simulink model "PositionControl_trajectory_obs"  (R2019a)
settings: Solver=ode3  StartTime=0.0  StopTime=100.0  FixedStep=Ts  RelTol=1e-3
values from neighbouring files (symbols this model uses):
  error_margin = 0.05    [Control_borroso_obstaculo_reference.m]    (also in Control_borroso_obstaculo_trajectory.m = 0)
  obsx = 3    [Control_borroso_obstaculo_reference.m]    (also in Control_borroso_obstaculo_trajectory.m = 2)
  obsy = 3    [Control_borroso_obstaculo_reference.m]    (also in Control_borroso_obstaculo_trajectory.m = 1)
  th_0 = w0    (= 0)    [Control_borroso_obstaculo_trajectory.m]
  Ts = 100e-3    (= 0.1)    [Control_borroso_obstaculo_reference.m]    (also in Control_borroso_obstaculo_trajectory.m)
  w0 = pi/2    (= 1.57079632679)    [Control_borroso_obstaculo_reference.m]    (also in Control_borroso_obstaculo_trajectory.m = 0)
  x0 = 0    [Control_borroso_obstaculo_reference.m]    (also in Control_borroso_obstaculo_trajectory.m = -5)
  x_0 = 0    [Control_borroso_obstaculo_trajectory.m]
  y0 = 0    [Control_borroso_obstaculo_reference.m]    (also in Control_borroso_obstaculo_trajectory.m)
  y_0 = y0    (= 0)    [Control_borroso_obstaculo_trajectory.m]
undefined symbols (not defined in the file or in its folder): DiscIntNeverNeededParam, sigbuilder_block
libraries: fuzblock x1, simulink x1
settings Model: Creator=mrblissfulgrin  LastModifiedBy=juanjosecordoba
settings DataIOCC: ReturnWorkspaceOutputs=off

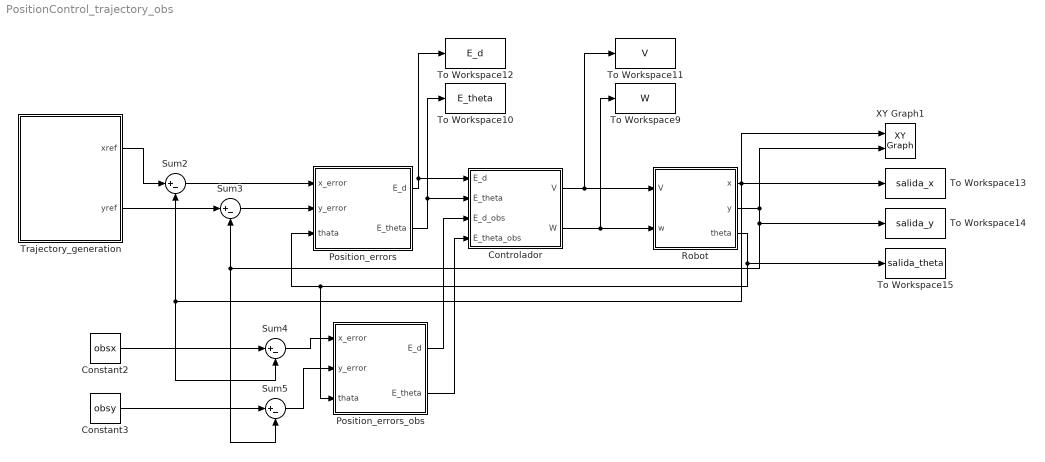
== system PositionControl_trajectory_obs ==
  Constant2 : Constant  Value=obsx  SampleTime=Ts
  Constant3 : Constant  Value=obsy  SampleTime=Ts
  Controlador : Subsystem
  Position_errors : Subsystem
  Position_errors_obs : Subsystem
  Robot : Subsystem
  Sum{2..5} (4 alike) : Sum  Inputs=|+-
  To Workspace10 : ToWorkspace  VariableName=E_theta  SaveFormat=Structure With Time  SampleTime=Ts
  To Workspace11 : ToWorkspace  VariableName=V  SaveFormat=Structure With Time  SampleTime=Ts
  To Workspace12 : ToWorkspace  VariableName=E_d  SaveFormat=Structure With Time  SampleTime=Ts
  To Workspace13 : ToWorkspace  VariableName=salida_x  SaveFormat=Structure With Time  SampleTime=Ts
  To Workspace14 : ToWorkspace  VariableName=salida_y  SaveFormat=Structure With Time  SampleTime=Ts
  To Workspace15 : ToWorkspace  VariableName=salida_theta  SaveFormat=Structure With Time  SampleTime=Ts
  To Workspace9 : ToWorkspace  VariableName=W  SaveFormat=Structure With Time  SampleTime=Ts
  Trajectory_generation : Subsystem
  XY Graph1 : simulink/Sinks/XY Graph  xmin=-10  xmax=10  ymin=-10  ymax=10  st=Ts
  wires:
  Constant3/1 -> Sum5/1
  Controlador/1("V ") -> Robot/1(V), To Workspace11/1
  Position_errors_obs/1(E_d) -> Controlador/3(E_d_obs)
  Position_errors/2(E_theta) -> To Workspace10/1, Controlador/2(E_theta)
  Trajectory_generation/2(yref) -> Sum3/1
  Constant2/1 -> Sum4/1
  Sum4/1 -> Position_errors_obs/1(x_error)
  Sum5/1 -> Position_errors_obs/2(y_error)
  Robot/3(theta) -> To Workspace15/1, Position_errors_obs/3(thata), Position_errors/3(thata)
  Controlador/2(W) -> To Workspace9/1, Robot/2(w)
  Robot/2(y) -> To Workspace14/1, Sum3/2, Sum5/2, XY Graph1/2
  Position_errors/1(E_d) -> Controlador/1("E_d "), To Workspace12/1
  Position_errors_obs/2(E_theta) -> Controlador/4(E_theta_obs)
  Robot/1(x) -> XY Graph1/1, To Workspace13/1, Sum4/2, Sum2/2
  Sum3/1 -> Position_errors/2(y_error)
  Trajectory_generation/1(xref) -> Sum2/1
  Sum2/1 -> Position_errors/1(x_error)

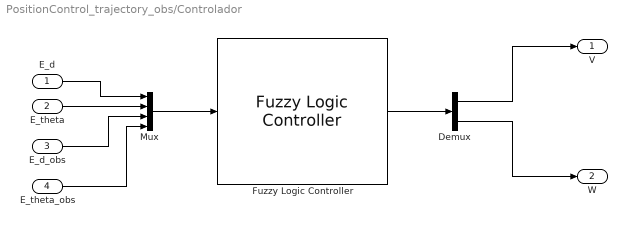
== system PositionControl_trajectory_obs/Controlador ==
  "E_d " : Inport  SampleTime=Ts
  E_theta : Inport  Port=2  SampleTime=Ts
  E_d_obs : Inport  Port=3  SampleTime=Ts
  E_theta_obs : Inport  Port=4  SampleTime=Ts
  Demux : Demux  Outputs=2
  Fuzzy Logic Controller : fuzblock/Fuzzy Logic  Controller  FIS=fis_name  OutputSampleNumber=101  DataType=double  FuzzifiedInputs=off  RuleFiringStrengths=off  RuleOutputs=off  AggregatedOutputs=off  SimulateUsing=Interpreted execution  OutOfRangeInputValueMessage=warning  NoRuleFiredMessage=warning  EmptyOutputFuzzySetMessage=warning
  Mux : Mux
  "V " : Outport  SampleTime=Ts
  W : Outport  Port=2  SampleTime=Ts
  wires:
  Demux/1 -> "V "/1
  Demux/2 -> W/1
  E_theta/1 -> Mux/2
  Mux/1 -> Fuzzy Logic Controller/1
  Fuzzy Logic Controller/1 -> Demux/1
  "E_d "/1 -> Mux/1
  E_d_obs/1 -> Mux/3
  E_theta_obs/1 -> Mux/4

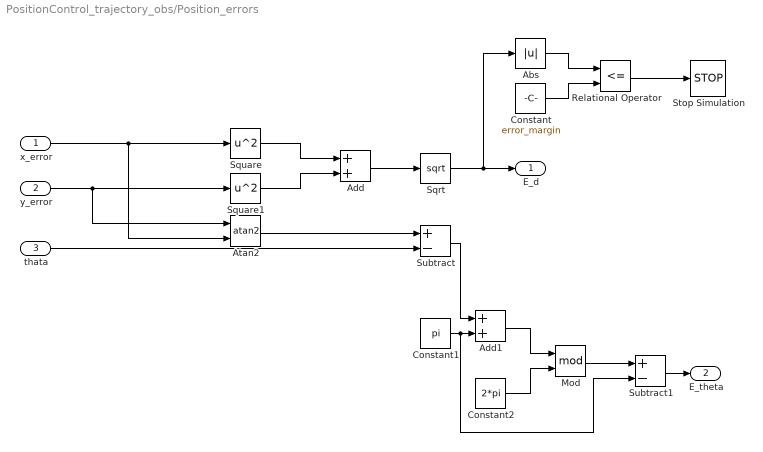
== system PositionControl_trajectory_obs/Position_errors ==
  x_error : Inport  SampleTime=Ts
  y_error : Inport  Port=2  SampleTime=Ts
  thata : Inport  Port=3  SampleTime=Ts
  Abs : Abs
  Add : Sum
  Add1 : Sum
  Atan2 : Trigonometry  Operator=atan2
  Constant : Constant  Value=error_margin  SampleTime=Ts
  Constant1 : Constant  Value=pi  SampleTime=Ts
  Constant2 : Constant  Value=2*pi
  Mod : Math  Operator=mod  SaturateOnIntegerOverflow=on
  Relational Operator : RelationalOperator  Operator=<=  OutDataTypeStr=boolean  RndMeth=Simplest
  Sqrt : Sqrt  SaturateOnIntegerOverflow=on
  Square : Math  Operator=square  SaturateOnIntegerOverflow=on
  Square1 : Math  Operator=square  SaturateOnIntegerOverflow=on
  Stop Simulation : Stop
  Subtract : Sum  Inputs=+-
  Subtract1 : Sum  Inputs=+-
  E_d : Outport  SampleTime=Ts
  E_theta : Outport  Port=2  SampleTime=Ts
  wires:
  Square/1 -> Add/1
  y_error/1 -> Square1/1, Atan2/1
  Add/1 -> Sqrt/1
  Square1/1 -> Add/2
  thata/1 -> Subtract/2
  x_error/1 -> Square/1, Atan2/2
  Subtract/1 -> Add1/1
  Atan2/1 -> Subtract/1
  Constant1/1 -> Subtract1/2, Add1/2
  Add1/1 -> Mod/1
  Constant2/1 -> Mod/2
  Mod/1 -> Subtract1/1
  Subtract1/1 -> E_theta/1
  Constant/1 -> Relational Operator/2
  Abs/1 -> Relational Operator/1
  Sqrt/1 -> Abs/1, E_d/1
  Relational Operator/1 -> Stop Simulation/1

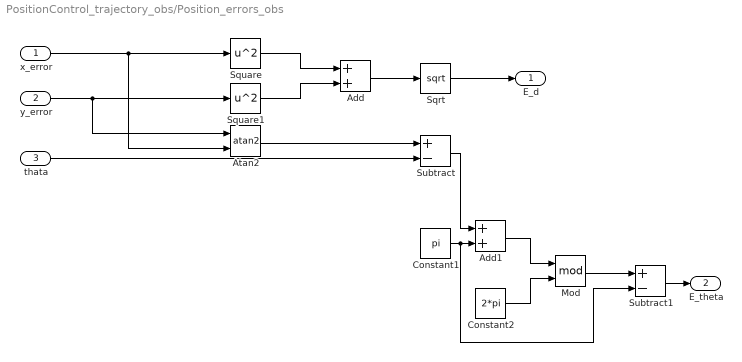
== system PositionControl_trajectory_obs/Position_errors_obs ==
  x_error : Inport  SampleTime=Ts
  y_error : Inport  Port=2  SampleTime=Ts
  thata : Inport  Port=3  SampleTime=Ts
  Add : Sum
  Add1 : Sum
  Atan2 : Trigonometry  Operator=atan2
  Constant1 : Constant  Value=pi  SampleTime=Ts
  Constant2 : Constant  Value=2*pi
  Mod : Math  Operator=mod  SaturateOnIntegerOverflow=on
  Sqrt : Sqrt  SaturateOnIntegerOverflow=on
  Square : Math  Operator=square  SaturateOnIntegerOverflow=on
  Square1 : Math  Operator=square  SaturateOnIntegerOverflow=on
  Subtract : Sum  Inputs=+-
  Subtract1 : Sum  Inputs=+-
  E_d : Outport  SampleTime=Ts
  E_theta : Outport  Port=2  SampleTime=Ts
  wires:
  Square/1 -> Add/1
  Sqrt/1 -> E_d/1
  y_error/1 -> Square1/1, Atan2/1
  Add/1 -> Sqrt/1
  Square1/1 -> Add/2
  thata/1 -> Subtract/2
  x_error/1 -> Square/1, Atan2/2
  Subtract/1 -> Add1/1
  Atan2/1 -> Subtract/1
  Constant1/1 -> Subtract1/2, Add1/2
  Add1/1 -> Mod/1
  Constant2/1 -> Mod/2
  Mod/1 -> Subtract1/1
  Subtract1/1 -> E_theta/1

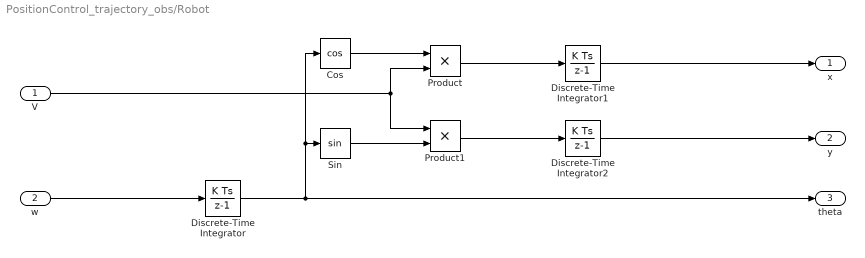
== system PositionControl_trajectory_obs/Robot ==
  V : Inport  SampleTime=Ts
  w : Inport  Port=2  SampleTime=Ts
  Cos : Trigonometry  Operator=cos
  Discrete-Time Integrator : DiscreteIntegrator  InitialCondition=w0  SampleTime=Ts  ICPrevOutput=DiscIntNeverNeededParam  ICPrevScaledInput=DiscIntNeverNeededParam
  Discrete-Time Integrator1 : DiscreteIntegrator  InitialCondition=x0  SampleTime=Ts  ICPrevOutput=DiscIntNeverNeededParam  ICPrevScaledInput=DiscIntNeverNeededParam
  Discrete-Time Integrator2 : DiscreteIntegrator  InitialCondition=y0  SampleTime=Ts  ICPrevOutput=DiscIntNeverNeededParam  ICPrevScaledInput=DiscIntNeverNeededParam
  Product : Product
  Product1 : Product
  Sin : Trigonometry
  x : Outport  SampleTime=Ts
  y : Outport  Port=2  SampleTime=Ts
  theta : Outport  Port=3  SampleTime=Ts
  wires:
  Discrete-Time Integrator2/1 -> y/1
  Product1/1 -> Discrete-Time Integrator2/1
  Cos/1 -> Product/1
  Sin/1 -> Product1/2
  w/1 -> Discrete-Time Integrator/1
  Discrete-Time Integrator1/1 -> x/1
  Product/1 -> Discrete-Time Integrator1/1
  V/1 -> Product/2, Product1/1
  Discrete-Time Integrator/1 -> theta/1, Sin/1, Cos/1

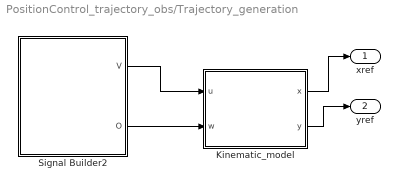
== system PositionControl_trajectory_obs/Trajectory_generation ==
  Kinematic_model : Subsystem
  Signal Builder2 : Subsystem  Tag=STV Subsys  LoadFcn=sigbuilder_block('load');  StartFcn=sigbuilder_block('start');  StopFcn=sigbuilder_block('stop');  ClipboardFcn=sigbuilder_block('clipboard');  mask(Sigbuilder block){tuvar=[0:10]}
      mask help: Sigbuilder GUI
      mask init:
      | if ~strcmp(get_param(bdroot(gcbh),'SimulationStatus'),'stopped') tuvar = sigbuilder_block('maskInit'); end
      settings: CopyFcn=sigbuilder_block('copy');  DeleteFcn=sigbuilder_block('delete');  ModelCloseFcn=sigbuilder_block('modelClose');  PreSaveFcn=sigbuilder_block('preSave');  PauseFcn=sigbuilder_block('pause')  ContinueFcn=sigbuilder_block('continue')  NameChangeFcn=sigbuilder_block('namechange');  OpenFcn=sigbuilder_block('open',[60 82.4 534.4 508 ]);  CloseFcn=sigbuilder_block('close');
      mask Display: plot(0, 0, 100, 100,[2, 2, 32, 32, 2], [68, 8, 8, 68, 68],[32, 2], [38, 38], [32, 19, 2],[53, 60, 44], [32, 17, 17, 2],[16, 16, 31, 31]);txt = getActiveGroup(gcbh);text(2, 100, txt,'verticalAlignment', 'top');
  xref : Outport
  yref : Outport  Port=2
  wires:
  Signal Builder2/1(V) -> Kinematic_model/1(u)
  Signal Builder2/2(O) -> Kinematic_model/2(w)
  Kinematic_model/1(x) -> xref/1
  Kinematic_model/2(y) -> yref/1

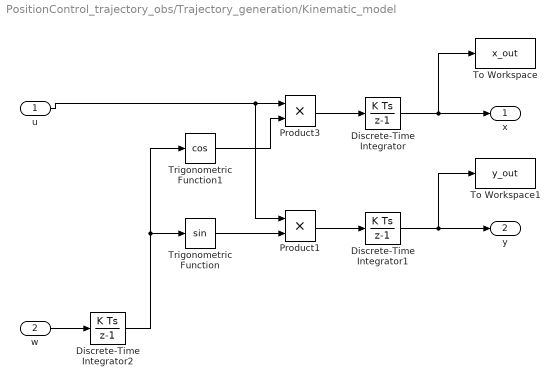
== system PositionControl_trajectory_obs/Trajectory_generation/Kinematic_model ==
  u : Inport
  w : Inport  Port=2
  Discrete-Time Integrator : DiscreteIntegrator  InitialCondition=x_0  SampleTime=Ts  ICPrevOutput=DiscIntNeverNeededParam  ICPrevScaledInput=DiscIntNeverNeededParam
  Discrete-Time Integrator1 : DiscreteIntegrator  InitialCondition=y_0  SampleTime=Ts  ICPrevOutput=DiscIntNeverNeededParam  ICPrevScaledInput=DiscIntNeverNeededParam
  Discrete-Time Integrator2 : DiscreteIntegrator  InitialCondition=th_0  SampleTime=Ts  ICPrevOutput=DiscIntNeverNeededParam  ICPrevScaledInput=DiscIntNeverNeededParam
  Product1 : Product
  Product3 : Product
  To Workspace : ToWorkspace  VariableName=x_out  SaveFormat=Structure With Time  SampleTime=Ts
  To Workspace1 : ToWorkspace  VariableName=y_out  SaveFormat=Structure With Time  SampleTime=Ts
  Trigonometric Function : Trigonometry
  Trigonometric Function1 : Trigonometry  Operator=cos
  x : Outport
  y : Outport  Port=2
  wires:
  Discrete-Time Integrator2/1 -> Trigonometric Function1/1, Trigonometric Function/1
  Product1/1 -> Discrete-Time Integrator1/1
  Product3/1 -> Discrete-Time Integrator/1
  w/1 -> Discrete-Time Integrator2/1
  Trigonometric Function/1 -> Product1/2
  u/1 -> Product1/1, Product3/1
  Trigonometric Function1/1 -> Product3/2
  Discrete-Time Integrator1/1 -> To Workspace1/1, y/1
  Discrete-Time Integrator/1 -> To Workspace/1, x/1

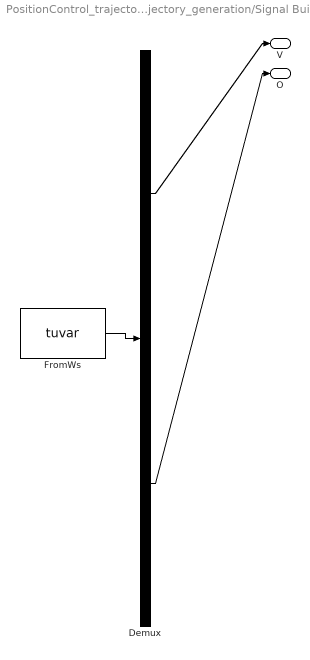
== system PositionControl_trajectory_obs/Trajectory_generation/Signal Builder2 ==
  Demux : Demux  Tag=STV Demux  Outputs=2
  FromWs : FromWorkspace  Tag=STV FromWs  VariableName=tuvar  SampleTime=0
      SigBuilderData=|
      | common.afterFinalStr = 'Extrapolate'
      | common.sampleTime = '0'
      | dataSet.timeRange = [0 115]
      | dataSet.name = 'Group 1'
      | sbobj.Groups.Name = 'Group 1'
      | sbobj.Groups.Signals(1).Name = 'V'
      | sbobj.Groups.Signals(1).XData = [0 87 87 115]
      | sbobj.Groups.Signals(1).YData = [0.25 0.25 0 0]
      | sbobj.Groups.Signals(2).Name = 'O'
      | sbobj.Groups.Signals(2).XData = [0 12 12 30.849 30.849 55.981 55.981 74.83 74.83 99.962 115]
      | sbobj.Groups.Signals(2).YData = [0 0 0.25 0.25 -0.25 -0.25 0.25 0.25 0 0 0]
      | sbobj.Groups.TimeRange = [0 115]
  V : Outport  Tag=STV Outport
  O : Outport  Tag=STV Outport  Port=2
  wires:
  FromWs/1 -> Demux/1
  Demux/1 -> V/1
  Demux/2 -> O/1
